simulink model "esercizio_1_massaMollaSmorzatore_2023b"  (R2023b)
settings: Solver=VariableStepAuto  StartTime=0.0  StopTime=20  RelTol=1e-3
PreLoadFcn:
  | % --------------------
  | % system's parameters:
  | % --------------------
  | 
  | M = 50 % massa
  | K = 0.02 % costante elastica
  | S = 0.02 % costante smorzatore
  | N = 5 % numero giunti intere molla
  | L = 10 % lunghezza giunti
  | 
  | % --------------------
  | % desired eigenvalues
  | % --------------------
  | 
  | eig_G = 1*[-1 -2 ]
  | 
  | % --------------------
  | % matrix and initial conditions
  | % --------------------
  | 
  | A = [   0     1    ;
  |       -K/M  -S/M   ]
  | 
  | 
  | B = [  0  ;
  |       1/M ]
  | 
  | 
  | C = [ 1 0 ;
  |       0 1 ]
  | 
  | D = zeros(size(C,1),size(B,2))
  | 
  | 
  | dimx = size(A,1)  % quindi dimx = 2
  | dimu = size(B,2)  % quindi dimu = 1
  | dimy = size(C,1)  % quindi dimy = 2
  | 
  | x0 = [20; % posizione iniziale
  |       100] % velocità iniziale
  | 
  | % --------------------
  | % certainty-equivalence state-feedback controller
  | % --------------------
  | 
  | G = place(A,B,eig_G) % costruisce matrice G dati gli autovalori desiderati
libraries: vrlib x14, sldrtlib x1
settings Model: Creator=39342  LastModifiedBy=simone
settings RTWCC: GPUComputeCapability=5.0

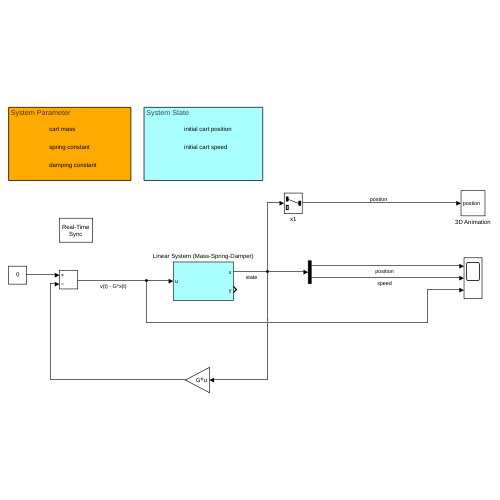
[thumbnail: Simulink's stored preview of the top-level diagram]
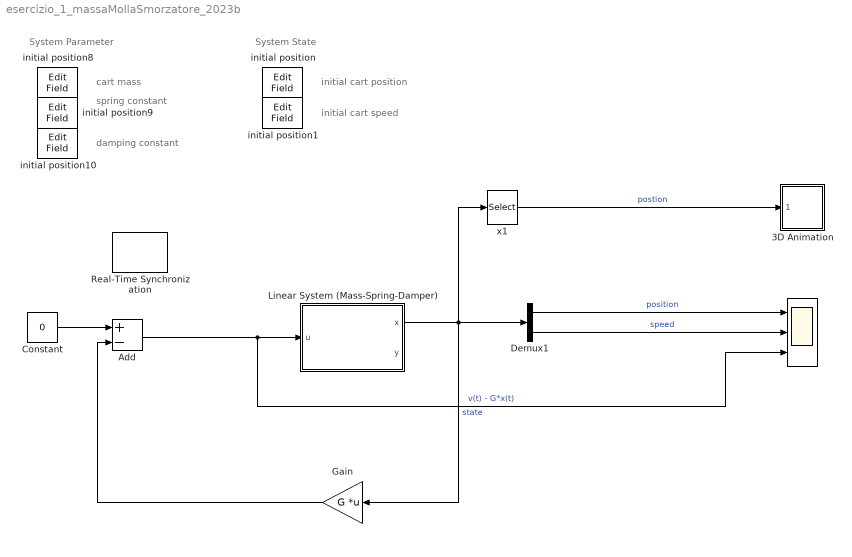
== system esercizio_1_massaMollaSmorzatore_2023b ==
  note: cart mass
  note: initial cart speed
  note: System State
  note: System Parameter
  note: spring constant
  note: initial cart position
  note: damping constant
  " " : Scope  NumInputPorts=3
  3D Animation : Subsystem
  Add : Sum  Inputs=+-
  Constant : Constant  Value=0
  Demux1 : Demux  Outputs=2
  Gain : Gain  Gain=G  Multiplication=Matrix(K*u)
  Linear System (Mass-Spring-Damper) : Subsystem
  Real-Time Synchronization : sldrtlib/Real-Time Synchronization  SampleTime=0.01  MaxMissedTicks=100  ShowMissedTicks=off  YieldWhenWaiting=off
  initial position{,1,8..10} (5 alike) : EditField  LabelPosition=Hide  ShowInitialText=on  Alignment=Center
  x1 : Selector  InputPortWidth=2  IndexOptions=Index vector (dialog)  Indices=[1]  OutputSizes=1
  wires:
  Gain/1 -> Add/2
  Constant/1 -> Add/1
  Add/1 -> Linear System (Mass-Spring-Damper)/1(u), " "/3  "v(t) - G*x(t)"
  Linear System (Mass-Spring-Damper)/1(x) -> x1/1, Demux1/1, Gain/1  "state"
  Demux1/2 -> " "/2  "speed"
  Demux1/1 -> " "/1  "position"
  x1/1 -> 3D Animation/1(postion)  "postion"

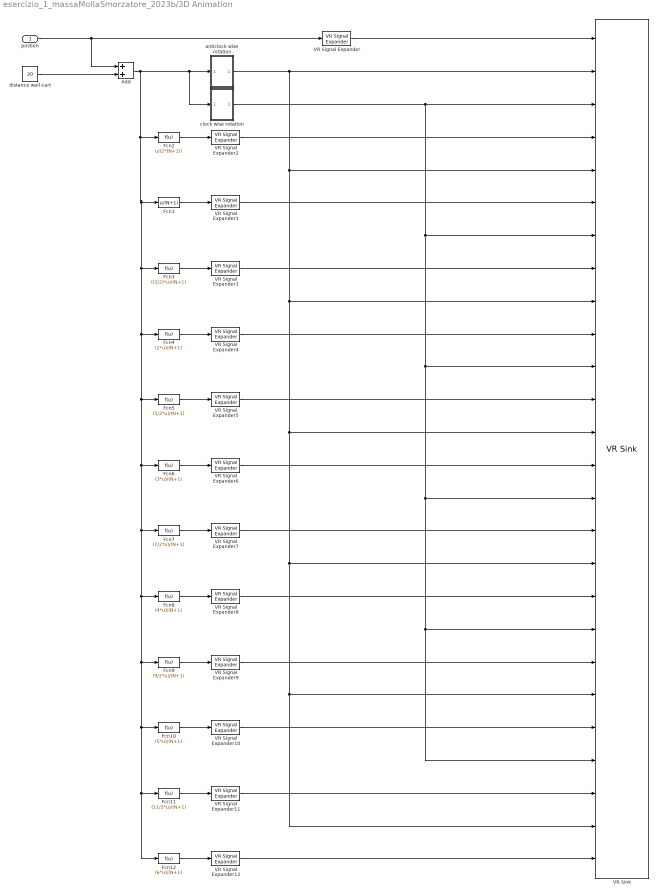
== system esercizio_1_massaMollaSmorzatore_2023b/3D Animation ==
  postion : Inport
  Add : Sum
  Fcn1 : Fcn  Expr=u/(N+1)
  Fcn10 : Fcn  Expr=(5*u)/(N+1)
  Fcn11 : Fcn  Expr=(11/2*u)/(N+1)
  Fcn12 : Fcn  Expr=(6*u)/(N+1)
  Fcn2 : Fcn  Expr=u/(2*(N+1))
  Fcn3 : Fcn  Expr=((3/2)*u)/(N+1)
  Fcn4 : Fcn  Expr=(2*u)/(N+1)
  Fcn5 : Fcn  Expr=(5/2*u)/(N+1)
  Fcn6 : Fcn  Expr=(3*u)/(N+1)
  Fcn7 : Fcn  Expr=(7/2*u)/(N+1)
  Fcn8 : Fcn  Expr=(4*u)/(N+1)
  Fcn9 : Fcn  Expr=(9/2*u)/(N+1)
  VR Signal Expander{,1..12} (13 alike) : vrlib/VR Signal Expander  outwidth=3  outidx=[1]
  VR Sink : vrlib/VR Sink  InstantiateOnLoad=on  SampleTime=0.1  ViewEnable=on  RemoteChange=off  RemoteView=off  FieldsWritten=cart.translation.3.1.1.double#joint_1.rotation.4.1.1.double#joint_2.rotation.4.1.1.double#joint_2.translation.3.1.1.double#joint_3.rotation.4.1.1.double#joint_3.translation.3.1.1.double#joint_4.rotation.4.1.1.double#joint_4.translation.3.1.1.double#joint_5.rotation.4.1.1.double#joint_5.translation.3.1.1.double#joint_6.rotation.4.1.1.double#joint_6.translation.3.1.1.double#joint_7.rotation.4.1.1.double#joint_7.translation.3.1.1.double#joint_8.rotation.4.1.1.double#joint_8.translation.3.1.1.double#joint_9.rotation.4.1.1.double#joint_9.translation.3.1.1.double#joint_10.rotation.4.1.1.double#joint_10.translation.3.1.1.double#joint_11.rotation.4.1.1.double#joint_11.translation.3.1.1.double#joint_12.rotation.4.1.1.double#joint_12.translation.3.1.1.double#joint_13.rotation.4.1.1.double#joint_13.translation.3.1.1.double  WorldFileName=animazioneCarrello.x3d  AutoView=on  VideoDimensions=[]  AllowVariableSize=off  FigureProperties="{'Position', 'Name', 'Viewpoint', 'CameraBound', 'CameraDirection', 'CameraPosition', 'CameraUpVector', 'ZoomFactor', 'Antialiasing', 'Headlight', 'Lighting', 'Sound', 'StatusBar', 'Stereo3D', 'Stereo3DCameraOffset', 'Stereo3DHIT', 'ToolBar', 'Textures', 'Transparency', 'Triad', 'Wireframe', 'NavZones', 'NavMode', 'NavSpeed', 'CaptureFileFormat', 'CaptureFileName', 'Record2DCompressMethod', 'Record2DCompressQuality', 'Record2D', 'Record2DFileName', 'Record2DFPS', 'NavPanel'; [1.3670000000000000e+03   1.2500000000000000e+02   1.4150000000000000e+03   9.0400000000000000e+02], '', 'frontal view', 'on', [0.0000000000000000e+00   0.0000000000000000e+00  -1.0000000000000000e+00], [0.0000000000000000e+00   0.0000000000000000e+00   3.7000000000000000e+01], [0.0000000000000000e+00   1.0000000000000000e+00   0.0000000000000000e+00], [1.0000000000000000e+00], 'on', 'on', 'on', 'on', 'on', 'off', [1.0000000149011612e-01], [0.0000000000000000e+00], 'on', 'on', 'on', 'none', 'off', 'off', 'fly', 'normal', 'tif', '%f_anim_%n.tif', 'auto', [7.5000000000000000e+01], 'off', '%f_anim_%n.avi', 'auto', 'halfbar'}"
  anticlock wise rotation : Subsystem
  clock wise rotation : Subsystem
  distance wall-cart : Constant  Value=20
  wires:
  postion/1 -> Add/1, VR Signal Expander/1
  distance wall-cart/1 -> Add/2
  Fcn2/1 -> VR Signal Expander2/1
  Fcn3/1 -> VR Signal Expander3/1
  Fcn4/1 -> VR Signal Expander4/1
  Fcn5/1 -> VR Signal Expander5/1
  Fcn6/1 -> VR Signal Expander6/1
  Fcn7/1 -> VR Signal Expander7/1
  Fcn8/1 -> VR Signal Expander8/1
  Fcn9/1 -> VR Signal Expander9/1
  VR Signal Expander/1 -> VR Sink/1
  anticlock wise rotation/1(Out1) -> VR Sink/25, VR Sink/21, VR Sink/17, VR Sink/13, VR Sink/9, VR Sink/5, VR Sink/2
  clock wise rotation/1(Out1) -> VR Sink/23, VR Sink/19, VR Sink/15, VR Sink/11, VR Sink/7, VR Sink/3
  VR Signal Expander2/1 -> VR Sink/4
  VR Signal Expander1/1 -> VR Sink/6
  VR Signal Expander3/1 -> VR Sink/8
  VR Signal Expander4/1 -> VR Sink/10
  VR Signal Expander5/1 -> VR Sink/12
  VR Signal Expander6/1 -> VR Sink/14
  VR Signal Expander7/1 -> VR Sink/16
  VR Signal Expander8/1 -> VR Sink/18
  VR Signal Expander9/1 -> VR Sink/20
  VR Signal Expander10/1 -> VR Sink/22
  Add/1 -> clock wise rotation/1(In1), anticlock wise rotation/1(In1), Fcn12/1, Fcn11/1, Fcn10/1, Fcn9/1, Fcn8/1, Fcn7/1, Fcn6/1, Fcn5/1, Fcn4/1, Fcn3/1, Fcn1/1, Fcn2/1
  Fcn10/1 -> VR Signal Expander10/1
  Fcn11/1 -> VR Signal Expander11/1
  VR Signal Expander11/1 -> VR Sink/24
  Fcn12/1 -> VR Signal Expander12/1
  VR Signal Expander12/1 -> VR Sink/26
  Fcn1/1 -> VR Signal Expander1/1

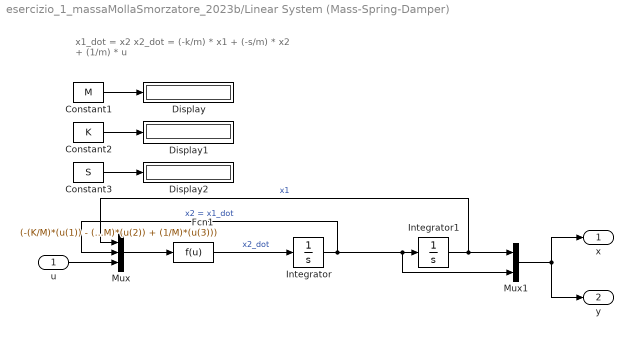
== system esercizio_1_massaMollaSmorzatore_2023b/Linear System (Mass-Spring-Damper) ==
  note: x1_dot = x2
      | x2_dot = (-k/m) * x1 + (-s/m) * x2 + (1/m) * u
  u : Inport
  Constant1 : Constant  Value=M
  Constant2 : Constant  Value=K
  Constant3 : Constant  Value=S
  Display : Display
  Display1 : Display
  Display2 : Display
  Fcn1 : Fcn  Expr=(-(K/M)*(u(1)) - (S/M)*(u(2)) + (1/M)*(u(3)))
  Integrator : Integrator  InitialCondition=x0(2)
  Integrator1 : Integrator  InitialCondition=x0(1)
  Mux : Mux  Inputs=3
  Mux1 : Mux  Inputs=2
  x : Outport
  y : Outport  Port=2
  wires:
  Fcn1/1 -> Integrator/1  "x2_dot"
  Integrator/1 -> Mux/2, Mux1/2, Integrator1/1  "x2 = x1_dot"
  Mux/1 -> Fcn1/1
  u/1 -> Mux/3
  Integrator1/1 -> Mux/1, Mux1/1  "x1"
  Mux1/1 -> x/1, y/1
  Constant2/1 -> Display1/1
  Constant3/1 -> Display2/1
  Constant1/1 -> Display/1

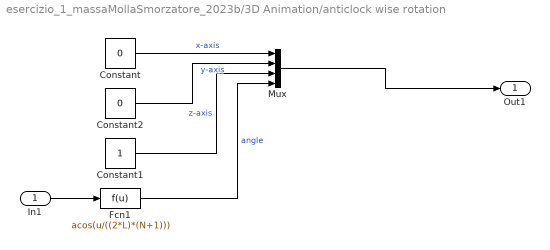
== system esercizio_1_massaMollaSmorzatore_2023b/3D Animation/anticlock wise rotation ==
  In1 : Inport
  Constant : Constant  Value=0
  Constant1 : Constant
  Constant2 : Constant  Value=0
  Fcn1 : Fcn  Expr=acos(u/((2*L)*(N+1)))
  Mux : Mux
  Out1 : Outport
  wires:
  Fcn1/1 -> Mux/4  "angle"
  Constant1/1 -> Mux/3  "z-axis"
  Constant2/1 -> Mux/2  "y-axis"
  Constant/1 -> Mux/1  "x-axis"
  In1/1 -> Fcn1/1
  Mux/1 -> Out1/1

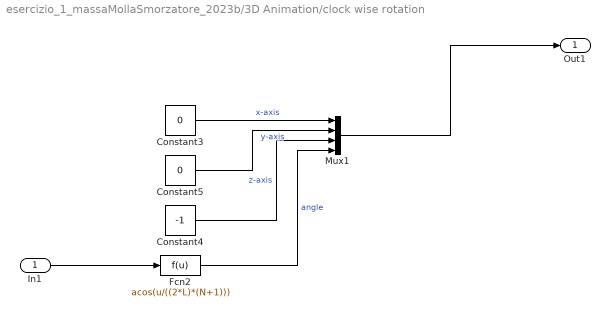
== system esercizio_1_massaMollaSmorzatore_2023b/3D Animation/clock wise rotation ==
  In1 : Inport
  Constant3 : Constant  Value=0
  Constant4 : Constant  Value=-1
  Constant5 : Constant  Value=0
  Fcn2 : Fcn  Expr=acos(u/((2*L)*(N+1)))
  Mux1 : Mux
  Out1 : Outport
  wires:
  Constant4/1 -> Mux1/3  "z-axis"
  Constant3/1 -> Mux1/1  "x-axis"
  Fcn2/1 -> Mux1/4  "angle"
  Constant5/1 -> Mux1/2  "y-axis"
  In1/1 -> Fcn2/1
  Mux1/1 -> Out1/1
